simulink model "ACT03"  (R2025a)
settings: Solver=VariableStepAuto  StartTime=0.0  StopTime=inf  RelTol=1e-3
settings Model: Creator=Juan Francisco Félix  LastModifiedBy=Juan Francisco Félix

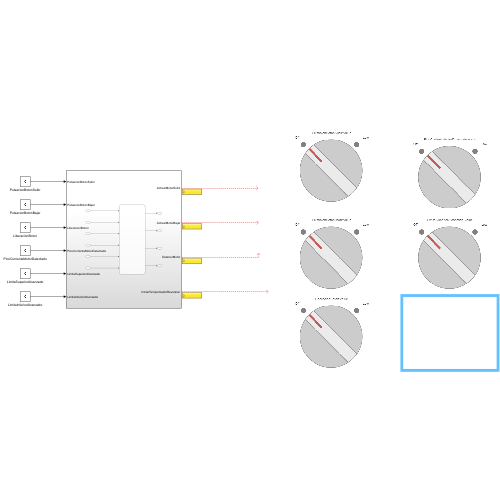
[thumbnail: Simulink's stored preview of the top-level diagram]
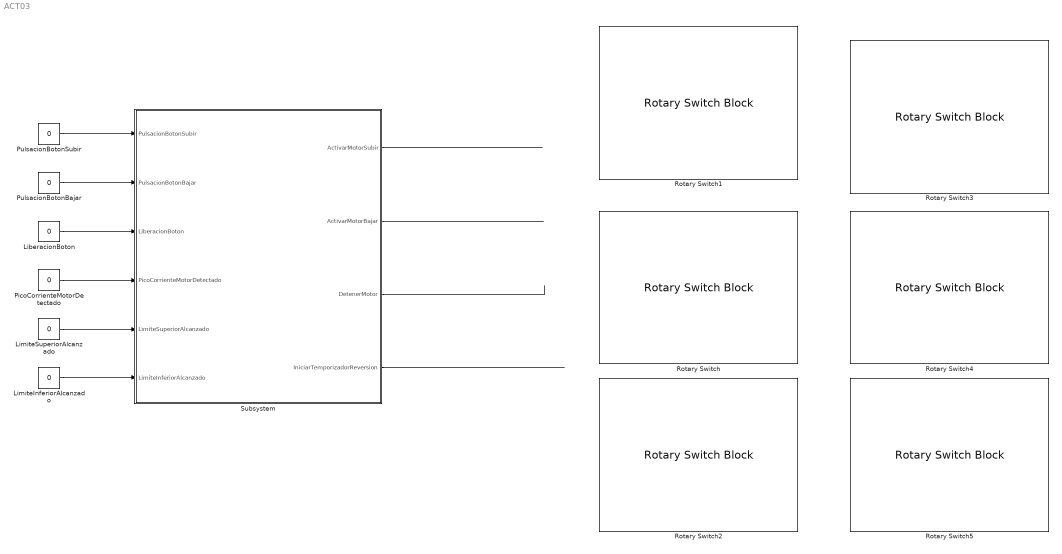
== system ACT03 ==
  LiberacionBoton : Constant  Value=0  OutDataTypeStr=uint8
  LimiteInferiorAlcanzado : Constant  Value=0  OutDataTypeStr=uint8
  LimiteSuperiorAlcanzado : Constant  Value=0  OutDataTypeStr=uint8
  PicoCorrienteMotorDetectado : Constant  Value=0  OutDataTypeStr=uint8
  PulsacionBotonBajar : Constant  Value=0  OutDataTypeStr=uint8
  PulsacionBotonSubir : Constant  Value=0  OutDataTypeStr=uint8
  Rotary Switch{,1..5} (6 alike) : RotarySwitchBlock
  Subsystem : Subsystem
  wires:
  LimiteInferiorAlcanzado/1 -> Subsystem/6(LimiteInferiorAlcanzado)
  LimiteSuperiorAlcanzado/1 -> Subsystem/5(LimiteSuperiorAlcanzado)
  PicoCorrienteMotorDetectado/1 -> Subsystem/4(PicoCorrienteMotorDetectado)
  LiberacionBoton/1 -> Subsystem/3(LiberacionBoton)
  PulsacionBotonBajar/1 -> Subsystem/2(PulsacionBotonBajar)
  PulsacionBotonSubir/1 -> Subsystem/1(PulsacionBotonSubir)
  Subsystem/1(ActivarMotorSubir) -> ?
  Subsystem/2(ActivarMotorBajar) -> ?
  Subsystem/3(DetenerMotor) -> ?
  Subsystem/4(IniciarTemporizadorReversion) -> ?

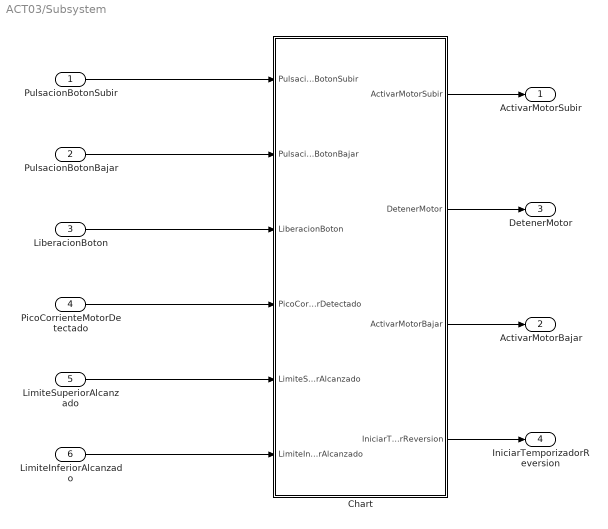
== system ACT03/Subsystem ==
  PulsacionBotonSubir : Inport  OutDataTypeStr=uint8
  PulsacionBotonBajar : Inport  Port=2  OutDataTypeStr=uint8
  LiberacionBoton : Inport  Port=3  OutDataTypeStr=uint8
  PicoCorrienteMotorDetectado : Inport  Port=4  OutDataTypeStr=uint8
  LimiteSuperiorAlcanzado : Inport  Port=5  OutDataTypeStr=uint8
  LimiteInferiorAlcanzado : Inport  Port=6  OutDataTypeStr=uint8
  Chart : Stateflow chart  TreatAsAtomicUnit=on
  ActivarMotorSubir : Outport  OutDataTypeStr=double
  ActivarMotorBajar : Outport  Port=2  OutDataTypeStr=double
  DetenerMotor : Outport  Port=3  OutDataTypeStr=double
  IniciarTemporizadorReversion : Outport  Port=4  OutDataTypeStr=double
  wires:
  PulsacionBotonBajar/1 -> Chart/2(PulsacionBotonBajar)
  LimiteSuperiorAlcanzado/1 -> Chart/5(LimiteSuperiorAlcanzado)
  PicoCorrienteMotorDetectado/1 -> Chart/4(PicoCorrienteMotorDetectado)
  LimiteInferiorAlcanzado/1 -> Chart/6(LimiteInferiorAlcanzado)
  PulsacionBotonSubir/1 -> Chart/1(PulsacionBotonSubir)
  LiberacionBoton/1 -> Chart/3(LiberacionBoton)
  Chart/1(ActivarMotorSubir) -> ActivarMotorSubir/1
  Chart/3(ActivarMotorBajar) -> ActivarMotorBajar/1
  Chart/2(DetenerMotor) -> DetenerMotor/1
  Chart/4(IniciarTemporizadorReversion) -> IniciarTemporizadorReversion/1

== stateflow chart ACT03/Subsystem/Chart ==
  state Subiendo
    during:
    ActivarMotorSubir= 1
    ActivarMotorBajar= 0
    DetenerMotor= 0
    IniciarTemporizadorReversion=0
  state Reposo
    during:
    ActivarMotorSubir= 0
    ActivarMotorBajar= 0
    DetenerMotor= 0
    IniciarTemporizadorReversion=0
  state Bajando
    during:
    ActivarMotorSubir= 0
    ActivarMotorBajar= 1
    DetenerMotor= 0
    IniciarTemporizadorReversion=0
  state Bloqueado
    during:
    ActivarMotorSubir= 0
    ActivarMotorBajar= 0
    DetenerMotor= 1
    IniciarTemporizadorReversion=1
  state Reversion
    during:
    ActivarMotorSubir= 0
    ActivarMotorBajar= 1
    DetenerMotor= 0
    IniciarTemporizadorReversion=0
  (default) -> Reposo
  Subiendo -> Bloqueado [order 2] : [PicoCorrienteMotorDetectado==1]
  Reposo -> Subiendo [order 1] : [PulsacionBotonSubir==1]
  Subiendo -> Reposo [order 1] : [(LiberacionBoton==1 && PulsacionBotonSubir==0)|| LimiteSuperiorAlcanzado]
  Reposo -> Bajando [order 2] : [PulsacionBotonBajar==1]
  Bajando -> Reposo : [(LiberacionBoton==1 & PulsacionBotonBajar==0)||LimiteInferiorAlcanzado==1]
  Bloqueado -> Reversion : [IniciarTemporizadorReversion==1]
  Reversion -> Reposo : [LimiteInferiorAlcanzado==1]
  data: PulsacionBotonSubir input; PulsacionBotonBajar input; LiberacionBoton input; PicoCorrienteMotorDetectado input; LimiteSuperiorAlcanzado input; LimiteInferiorAlcanzado input; ActivarMotorSubir output; DetenerMotor output; ActivarMotorBajar output; IniciarTemporizadorReversion output
